simulink model "HeatXTest2D"  (R2015a)
settings: Solver=FixedStepDiscrete  StartTime=0.0  StopTime=tsim  FixedStep=dt  RelTol=1e-3
values from neighbouring files (symbols this model uses):
  Cp1d = Cp*ones(length(y0),1)'    [run_HeatXTest2D.m]
  Cp2d = Cp*ones(length(y0),length(x))    [run_HeatXTest2D.m]
  hb = 0.03    [run_HeatXTest2D.m]
  ht = 0.03    [run_HeatXTest2D.m]
  k1d = k*ones(length(y0),1)'    [run_HeatXTest2D.m]
  k2d = k*ones(length(y0),length(x))    [run_HeatXTest2D.m]
  n = length(x)    [run_HeatXTest2D.m]
  rho1d = rho*ones(length(y0),1)'    [run_HeatXTest2D.m]
  rho2d = rho*ones(length(y0),length(x))    [run_HeatXTest2D.m]
  Tb = 800    [run_HeatXTest2D.m]
  Tt = 650    [run_HeatXTest2D.m]
libraries: lib_Conduction_HeatX1DVarPropsAndGenBCs x1, lib_Conduction_2DCondADI x1
settings Model: Creator=jlkratz  LastModifiedBy=jlkratz

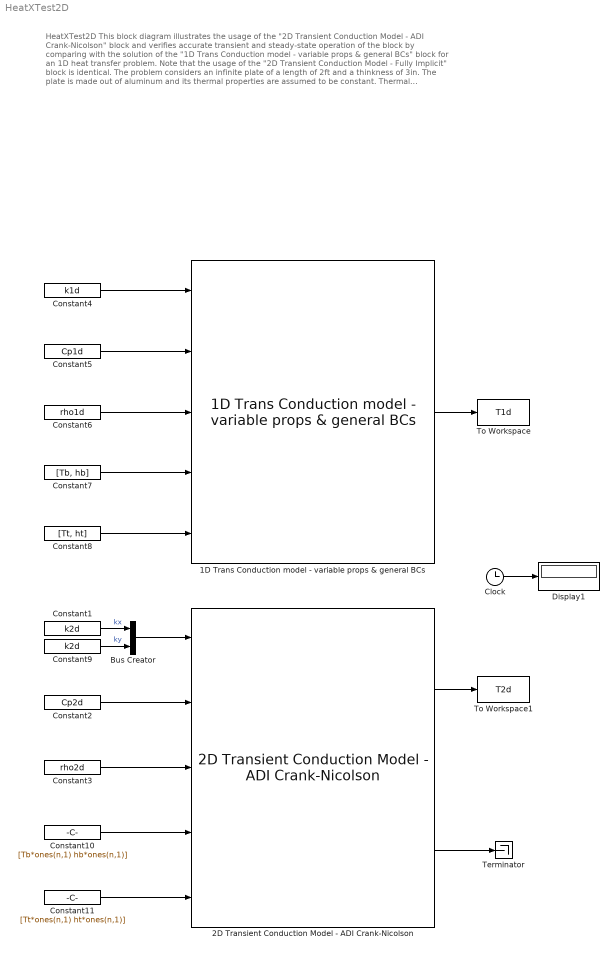
== system HeatXTest2D ==
  note: HeatXTest2D
      |
      | This block diagram illustrates the usage of the "2D Transient Conduction Model - ADI Crank-Nicolson" block
      | and verifies accurate transient and steady-state operation of the block by comparing with the solution of the "1D Trans
      | Conduction model - variable props & general BCs" block for an 1D heat transfer problem. Note that the usage of the
      | "2D Transient Conduction Model - Fully Implicit" block is identical.
      |
      | The problem considers an infinite plate of a length of 2ft and a thinkness of 3in. The plate is made out of aluminum and
      | its thermal properties are assumed to be constant.
      | Thermal conductivity, k = 0.0328Btu/(sec-ft-R)
      | Heat capacity, Cp = 6.92Btu/(slug-R)
      | Density, rho = 5.24slug/ft^3
      | The plate is at an initial temperature of 550R throughout. It is heated on the bottom surface by convection with a fluid
      | temperature of 800R and heat transfer coefficient of 0.03Btu/(sec-ft^2-R). It is heated on the top surface by convection
      | with a fluid temperature of 650R and heat transfer coefficient of 0.03Btu/(sec-ft^2-R)
  1D Trans Conduction model - variable props & general BCs : lib_Conduction_HeatX1DVarPropsAndGenBCs/1D Trans Conduction model - variable props & general BCs  x_M=y0  T0_M=T01d  dt_M=dt  a_M=off  convin_M=on  radin_M=off  condin_M=off  convout_M=on  radout_M=off  condout_M=off  BN_M=double(gcb)
  2D Transient Conduction Model - ADI Crank-Nicolson : lib_Conduction_2DCondADI/2D Transient Conduction Model - ADI Crank-Nicolson  T0_M=T02d  dt_M=dt  x_M=x  y_M=y0  shape_M=Planar in both directions  convL_M=off  radL_M=off  condL_M=off  convR_M=off  radR_M=off  condR_M=off  convB_M=on  radB_M=off  condB_M=off  convT_M=on  radT_M=off  condT_M=off  BN_M=double(gcb)
  Bus Creator : BusCreator  Inputs=2
  Clock : Clock
  Constant1 : Constant  Value=k2d
  Constant10 : Constant  Value=[Tb*ones(n,1) hb*ones(n,1)]
  Constant11 : Constant  Value=[Tt*ones(n,1) ht*ones(n,1)]
  Constant2 : Constant  Value=Cp2d
  Constant3 : Constant  Value=rho2d
  Constant4 : Constant  Value=k1d
  Constant5 : Constant  Value=Cp1d
  Constant6 : Constant  Value=rho1d
  Constant7 : Constant  Value=[Tb, hb]
  Constant8 : Constant  Value=[Tt, ht]
  Constant9 : Constant  Value=k2d
  Display1 : Display
  Terminator : Terminator
  To Workspace : ToWorkspace  VariableName=T1d  SaveFormat=Timeseries  SampleTime=-1
  To Workspace1 : ToWorkspace  VariableName=T2d  SaveFormat=Timeseries  SampleTime=-1
  wires:
  Constant1/1 -> Bus Creator/1  "kx"
  Constant9/1 -> Bus Creator/2  "ky"
  Bus Creator/1 -> 2D Transient Conduction Model - ADI Crank-Nicolson/1
  Constant4/1 -> 1D Trans Conduction model - variable props & general BCs/1
  Constant5/1 -> 1D Trans Conduction model - variable props & general BCs/2
  Constant6/1 -> 1D Trans Conduction model - variable props & general BCs/3
  Constant2/1 -> 2D Transient Conduction Model - ADI Crank-Nicolson/2
  Constant3/1 -> 2D Transient Conduction Model - ADI Crank-Nicolson/3
  Constant7/1 -> 1D Trans Conduction model - variable props & general BCs/4
  Constant8/1 -> 1D Trans Conduction model - variable props & general BCs/5
  Constant11/1 -> 2D Transient Conduction Model - ADI Crank-Nicolson/5
  Constant10/1 -> 2D Transient Conduction Model - ADI Crank-Nicolson/4
  1D Trans Conduction model - variable props & general BCs/1 -> To Workspace/1
  2D Transient Conduction Model - ADI Crank-Nicolson/1 -> To Workspace1/1
  2D Transient Conduction Model - ADI Crank-Nicolson/2 -> Terminator/1
  Clock/1 -> Display1/1
